simulink model "DroneSimulation"  (R2024a)
settings: Solver=VariableStepAuto  StartTime=0.0  StopTime=100  MaxStep=1e-4  MinStep=1e-6  RelTol=1e-3
undefined symbols (not defined in the file or in its folder): crot, d, g, gustX, gustY, gustZ, I, I_inv, IMU, Ix, Iy, Iz, ks, kt, l, m, ms_mat_inv, pitch_max, rho, roll_max, w_max, windX, windY, windZ, X, Y, Z
libraries: sm_lib x25, nesl_utility x14, simulink x11, slctrl_autotuning x8, mpclib x1, matrix_library x1
(part 1 of 3)
settings Model: SimulationMode=accelerator  Creator=OBWELUC  LastModifiedBy=OBWELUC
settings RTWCC: GPUComputeCapability=3.5
settings ExplorerConfigSet: InternalSimMechanicsExplorerSettings="<ExplorerConfiguration><canonicalview>default</canonicalview><AnimationSetting><BasePlaybackSpeed>1.0</BasePlaybackSpeed><PlaybackSpeedFactor>1.0</PlaybackSpeedFactor></AnimationSetting><TilePanel><TileInfo><Tiles Columns=\"2\" Count=\"4\" Rows=\"2\"><Column Weight=\"0.5\"/><Column Weight=\"0.5\"/><Row Weight=\"0.5\"/><Row Weight=\"0.5\"/><Tile Height=\"1\" Width=\"1\" X=\"0\" Y=\"0\"/><Tile Height=\"1\" Width=\"1\" X=\"0\" Y=\"1\"/><Tile Height=\"1\" Width=\"1\" X=\"1\" Y=\"0\"/><Tile Height=\"1\" Width=\"1\" X=\"1\" Y=\"1\"/></Tiles></TileInfo><SceneInfo><SceneViewer><BGColor><R>0</R><G>0.60000002384185791</G><B>1</B></BGColor><Camera><DoPerspective>off</DoPerspective><Position><X>-0.126727844040819326</X><Y>-7.10861089777495625</Y><Z>0.564557807287776714</Z></Position><Center><X>-0.126727844040819326</X><Y>1.66442092997096287e-07</Y><Z>0.564557807287776714</Z></Center><Up><X>0</X><Y>-0</Y><Z>1</Z></Up><ViewLimDist>1</ViewLimDist><YLim>0.592155844887899185</YLim><XLim>1.20086496625296957</XLim></Camera></SceneViewer><SceneViewer><BGColor><R>0</R><G>0.60000002384185791</G><B>1</B></BGColor><Camera><DoPerspective>off</DoPerspective><Position><X>-0.0834409949380843785</X><Y>0.128196391023159995</Y><Z>6.64461915986203699</Z></Position><Center><X>-0.0834409949380843785</X><Y>0.128196391023159995</Y><Z>-0.000826375150197122821</Z></Center><Up><X>0</X><Y>1</Y><Z>-0</Z></Up><ViewLimDist>1</ViewLimDist><YLim>1.06033933028744309</YLim><XLim>2.1503196583719939</XLim></Camera></SceneViewer><SceneViewer><BGColor><R>0</R><G>0.60000002384185791</G><B>1</B></BGColor><Camera><DoPerspective>off</DoPerspective><Position><X>7.10861089448633621</X><Y>0.203267557456647152</Y><Z>0.620697073756145024</Z></Position><Center><X>-3.2395406890373124e-07</X><Y>0.203267557456647152</Y><Z>0.620697073756145024</Z></Center><Up><X>-0</X><Y>0</Y><Z>1</Z></Up><ViewLimDist>1</ViewLimDist><YLim>0.63905302021013588</YLim><XLim>1.29597029257354102</XLim></Camera></SceneViewer><SceneViewer><BGColor><R>0</R><G>0.60000002384185791</G><B>1</B></BGColor><Camera><DoPerspective>off</DoPerspective><Position><X>4.87676778458632754</X><Y>-4.76365474719023041</Y><Z>1.81715889286770405</Z></Position><Center><X>-0.476731396941828978</X><Y>0.432045443382936933</Y><Z>0.387933409665207618</Z></Center><Up><X>-0.133906028563009039</X><Y>0.132192075511948781</Y><Z>0.982137684179934967</Z></Up><ViewLimDist>1</ViewLimDist><YLim>1.82629377901128631</YLim><XLim>3.70364024307752571</XLim></Camera></SceneViewer></SceneInfo></TilePanel><MechEditorPanel><Cameras/><GfxPanelCameraMap/><VideoCreator><PlaybackSpeedRatio>1.2</PlaybackSpeedRatio><FrameRate>60</FrameRate><VideoFormat>MPEG-4</VideoFormat><FrameSize>[1280 720]</FrameSize></VideoCreator></MechEditorPanel></ExplorerConfiguration>"

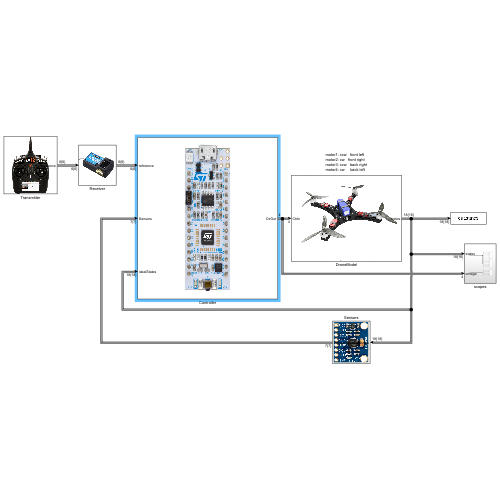
[thumbnail: Simulink's stored preview of the top-level diagram]
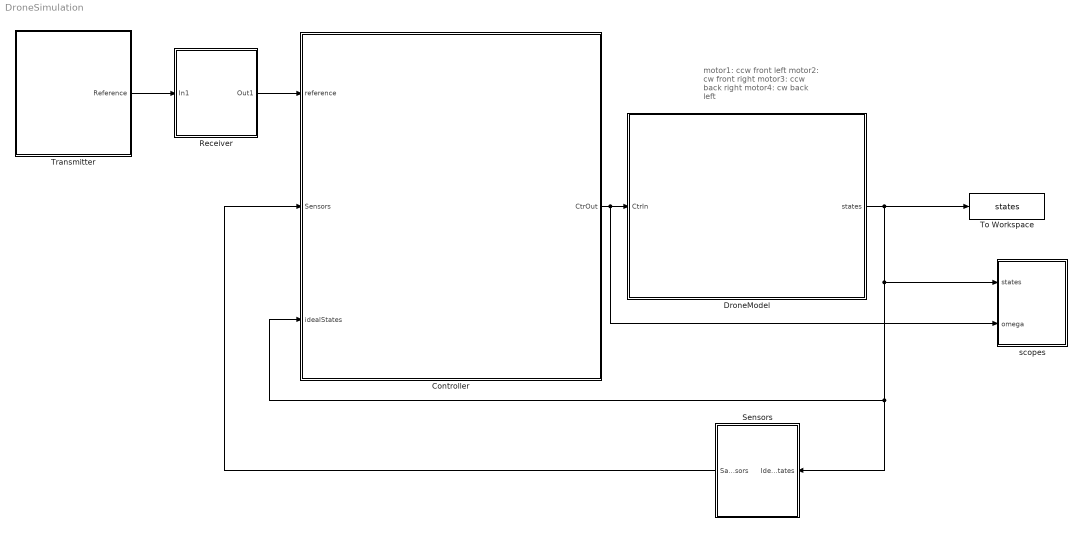
== system DroneSimulation ==
  note: motor1: ccw   front left
      | motor2: cw   front right
      | motor3: ccw   back right
      | motor4: cw     back left
  Controller : Subsystem
      mask Display: image('MFG_NUCLEO-L412KB.jpg');
  DroneModel : Subsystem
      mask Display: image('Assembly2.png');
  Receiver : Subsystem
      mask Display: image('$imagefile'); % Use "Edit Image" on toolstrip to change.
  Sensors : Subsystem
      mask Display: image('$imagefile'); % Use "Edit Image" on toolstrip to change.
  To Workspace : ToWorkspace  VariableName=states  SaveFormat=Timeseries  SampleTime=0.001
  Transmitter : Subsystem
      mask Display: image('$imagefile'); % Use "Edit Image" on toolstrip to change.
  scopes : Subsystem
  wires:
  DroneModel/1(states) -> To Workspace/1, scopes/1(states), Controller/3(idealStates), Sensors/1(IdealStates)
  Controller/1(CtrOut) -> scopes/2(omega), DroneModel/1(CtrIn)
  Transmitter/1(Reference) -> Receiver/1(In1)
  Receiver/1(Out1) -> Controller/1(reference)
  Sensors/1(SampeldSensors) -> Controller/2(Sensors)

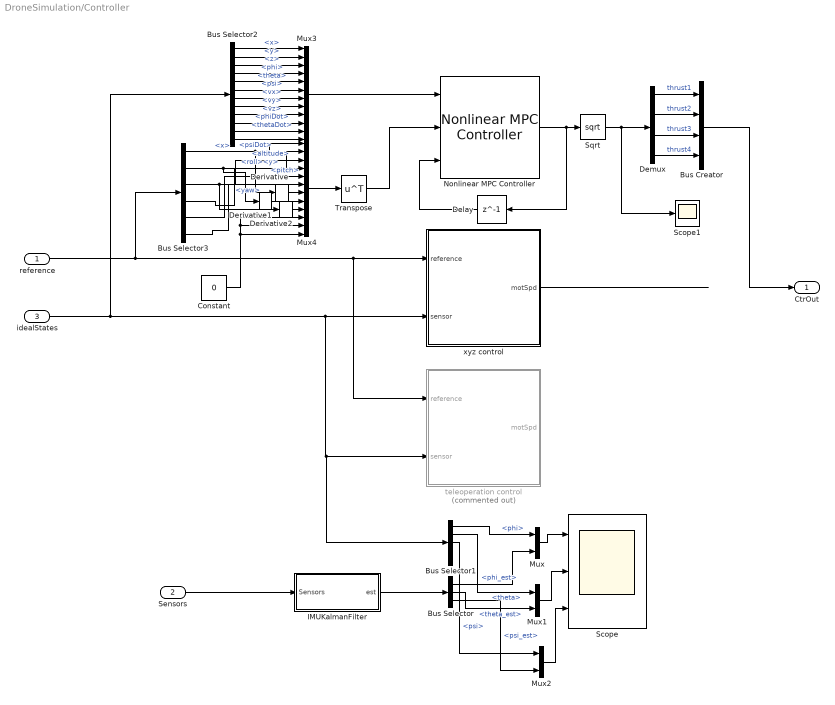
== system DroneSimulation/Controller ==
  reference : Inport
  Sensors : Inport  Port=2
  idealStates : Inport  Port=3
  Bus Creator : BusCreator  Inputs=4
  Bus Selector : BusSelector  OutputSignals=phi_est,theta_est,psi_est
  Bus Selector1 : BusSelector  OutputSignals=phi,theta,psi,ax,ay
  Bus Selector2 : BusSelector  OutputSignals=x,y,z,phi,theta,psi,vx,vy,vz,phiDot,thetaDot,psiDot
  Bus Selector3 : BusSelector  OutputSignals=x,y,altitude,roll,pitch,yaw
  Constant : Constant  Value=0
  Delay : Delay  DelayLength=1
  Demux : Demux
  Derivative : Derivative
  Derivative1 : Derivative
  Derivative2 : Derivative
  IMUKalmanFilter : Subsystem
  Mux : Mux  Inputs=2
  Mux1 : Mux  Inputs=2
  Mux2 : Mux  Inputs=2
  Mux3 : Mux  Inputs=12
  Mux4 : Mux  Inputs=12
  Nonlinear MPC Controller : mpclib/Nonlinear MPC Controller  nlmpcobj=nlmpcobj  UseObjectTs=on  UseMEX=off  md_enabled=off  mvtarget_enabled=off  param_enabled=off  cost_enabled=off  mvseq_enabled=off  stateseq_enabled=off  ovseq_enabled=off  slack_enabled=off  status_enabled=off  ov_min=off  ov_max=off  mv_min=off  mv_max=off  mvrate_min=off  mvrate_max=off  state_min=off  state_max=off  ov_weight=off  mv_weight=off  mvrate_weight=off  ecr_weight=off  nlp_initialize=off
  Scope : Scope  NumInputPorts=3
  Scope1 : Scope
  Sqrt : Sqrt
  Transpose : Math  Operator=transpose
  teleoperation control : Subsystem  Commented=on
  xyz control : Subsystem
  CtrOut : Outport
  wires:
  reference/1 -> Bus Selector3/1, teleoperation control/1(reference), xyz control/1(reference)
  xyz control/1(motSpd) -> ?
  IMUKalmanFilter/1(est) -> Bus Selector/1
  Bus Selector1/1 -> Mux/1  "<phi>"
  Bus Selector/1 -> Mux/2  "<phi_est>"
  Mux/1 -> Scope/1
  Mux1/1 -> Scope/2
  Bus Selector/2 -> Mux1/2  "<theta_est>"
  Bus Selector1/2 -> Mux1/1  "<theta>"
  idealStates/1 -> Bus Selector1/1, teleoperation control/2(sensor), xyz control/2(sensor), Bus Selector2/1
  Sensors/1 -> IMUKalmanFilter/1(Sensors)
  Bus Selector/3 -> Mux2/2  "<psi_est>"
  Bus Selector1/3 -> Mux2/1  "<psi>"
  Mux2/1 -> Scope/3
  Bus Selector2/1 -> Mux3/1  "<x>"
  Bus Selector2/2 -> Mux3/2  "<y>"
  Bus Selector2/3 -> Mux3/3  "<z>"
  Bus Selector2/4 -> Mux3/4  "<phi>"
  Bus Selector2/5 -> Mux3/5  "<theta>"
  Bus Selector2/6 -> Mux3/6  "<psi>"
  Bus Selector2/7 -> Mux3/7  "<vx>"
  Bus Selector2/8 -> Mux3/8  "<vy>"
  Bus Selector2/9 -> Mux3/9  "<vz>"
  Bus Selector2/10 -> Mux3/10  "<phiDot>"
  Bus Selector2/11 -> Mux3/11  "<thetaDot>"
  Bus Selector2/12 -> Mux3/12  "<psiDot>"
  Mux3/1 -> Nonlinear MPC Controller/1
  Mux4/1 -> Transpose/1
  Bus Selector3/1 -> Derivative/1, Mux4/1  "<x>"
  Bus Selector3/2 -> Derivative1/1, Mux4/2  "<y>"
  Bus Selector3/3 -> Derivative2/1, Mux4/3  "<altitude>"
  Constant/1 -> Mux4/12, Mux4/11, Mux4/10
  Bus Selector3/4 -> Mux4/4  "<roll>"
  Bus Selector3/5 -> Mux4/5  "<pitch>"
  Bus Selector3/6 -> Mux4/6  "<yaw>"
  Delay/1 -> Nonlinear MPC Controller/3
  Nonlinear MPC Controller/1 -> Delay/1, Sqrt/1
  Demux/1 -> Bus Creator/1  "thrust1"
  Demux/2 -> Bus Creator/2  "thrust2"
  Demux/3 -> Bus Creator/3  "thrust3"
  Demux/4 -> Bus Creator/4  "thrust4"
  Bus Creator/1 -> CtrOut/1
  Transpose/1 -> Nonlinear MPC Controller/2
  Derivative/1 -> Mux4/7
  Derivative1/1 -> Mux4/8
  Derivative2/1 -> Mux4/9
  Sqrt/1 -> Scope1/1, Demux/1

== system DroneSimulation/DroneModel ==
  CtrIn : Inport
  ComputeThrust : Subsystem
  ComputeTorques : Subsystem
  Dynamics : Subsystem
  visualization : Subsystem
  states : Outport
  wires:
  CtrIn/1 -> ComputeThrust/1(omega), ComputeTorques/1(omega)
  ComputeThrust/1(Fz) -> Dynamics/1(Fz)  "fz"
  Dynamics/1(states) -> visualization/1(states), states/1
  ComputeTorques/1(tau) -> Dynamics/2(tau)  "tau"
  Dynamics/2(t) -> visualization/2(t)
  Dynamics/3(wind) -> visualization/3(wind)

== system DroneSimulation/Receiver ==
  In1 : Inport
  Out1 : Outport
  wires:
  In1/1 -> Out1/1

== system DroneSimulation/Sensors ==
  IdealStates : Inport
  Accelerometer : Subsystem
  Bus Creator : BusCreator  Inputs=3
  barometer : Subsystem
  gyroscope : Subsystem
  SampeldSensors : Outport
  wires:
  IdealStates/1 -> barometer/1(IdealStates), gyroscope/1(IdealStates), Accelerometer/1(IdealStates)
  Bus Creator/1 -> SampeldSensors/1
  Accelerometer/1(accelerometerStates) -> Bus Creator/3  "accelerometer"
  gyroscope/1(gyroscopeStates) -> Bus Creator/2  "gyroscope"
  barometer/1(barometerStates) -> Bus Creator/1  "barometer"

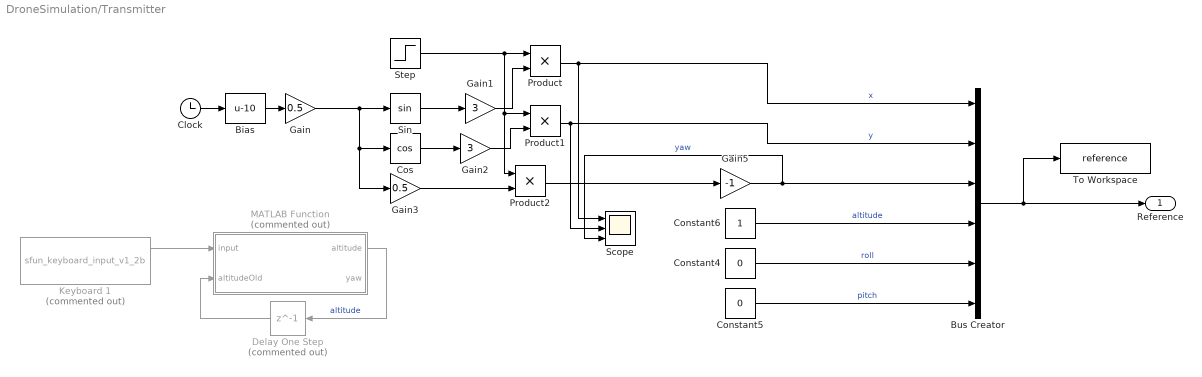
== system DroneSimulation/Transmitter ==
  Bias : Bias  Bias=-10  SaturateOnIntegerOverflow=off
  Bus Creator : BusCreator  Inputs=6
  Clock : Clock
  Constant4 : Constant  Value=0
  Constant5 : Constant  Value=0
  Constant6 : Constant
  Cos : Trigonometry  Operator=cos
  Delay One Step : Delay  Commented=on  DelayLength=1
  Gain : Gain  Gain=0.5
  Gain1 : Gain  Gain=3
  Gain2 : Gain  Gain=3
  Gain3 : Gain  Gain=0.5
  Gain5 : Gain  Gain=-1
  Keyboard 1 : M-S-Function  Commented=on  FunctionName=sfun_keyboard_input_v1_2b  mask(Keyboard Input){}
      mask help: Keyboard Input
      mask Display: fprintf('Keyboard');
  MATLAB Function : MATLAB Function  Commented=on  TreatAsAtomicUnit=on
  Product : Product
  Product1 : Product
  Product2 : Product
  Scope : Scope  NumInputPorts=3
  Sin : Trigonometry
  Step : Step  Time=10  SampleTime=0
  To Workspace : ToWorkspace  VariableName=reference  SaveFormat=Timeseries  SampleTime=0.001
  Reference : Outport
  wires:
  Bus Creator/1 -> To Workspace/1, Reference/1
  Product2/1 -> Gain5/1
  Cos/1 -> Gain2/1
  Sin/1 -> Gain1/1
  MATLAB Function/1(altitude) -> Delay One Step/1  "altitude"
  Constant4/1 -> Bus Creator/5  "roll"
  Constant5/1 -> Bus Creator/6  "pitch"
  Keyboard 1/1 -> MATLAB Function/1(input)
  Delay One Step/1 -> MATLAB Function/2(altitudeOld)
  Constant6/1 -> Bus Creator/4  "altitude"
  Clock/1 -> Bias/1
  Gain/1 -> Gain3/1, Cos/1, Sin/1
  Product/1 -> Scope/1, Bus Creator/1  "x"
  Product1/1 -> Scope/2, Bus Creator/2  "y"
  Gain1/1 -> Product/2
  Step/1 -> Product2/1, Product1/1, Product/1
  Gain2/1 -> Product1/2
  Gain5/1 -> Scope/3, Bus Creator/3  "yaw"
  Gain3/1 -> Product2/2
  Bias/1 -> Gain/1

== system DroneSimulation/scopes ==
  states : Inport
  omega : Inport  Port=2
  Bus Selector : BusSelector  OutputSignals=x,y,z,vx,vy,vz
  Bus Selector1 : BusSelector  OutputSignals=phi,theta,psi,phiDot,thetaDot,psiDot
  Bus Selector2 : BusSelector  OutputSignals=thrust1,thrust2,thrust3,thrust4
  Scope : Scope  NumInputPorts=4
  linearStates : Scope  NumInputPorts=6
  rotationalStates : Scope  NumInputPorts=6
  wires:
  states/1 -> Bus Selector1/1, Bus Selector/1
  Bus Selector1/1 -> rotationalStates/1  "<phi>"
  Bus Selector1/2 -> rotationalStates/2  "<theta>"
  Bus Selector1/3 -> rotationalStates/3  "<psi>"
  Bus Selector1/6 -> rotationalStates/6  "<psiDot>"
  Bus Selector1/4 -> rotationalStates/4  "<phiDot>"
  Bus Selector1/5 -> rotationalStates/5  "<thetaDot>"
  Bus Selector/2 -> linearStates/2  "<y>"
  Bus Selector/1 -> linearStates/1  "<x>"
  Bus Selector/3 -> linearStates/3  "<z>"
  Bus Selector/4 -> linearStates/4  "<vx>"
  Bus Selector/6 -> linearStates/6  "<vz>"
  Bus Selector/5 -> linearStates/5  "<vy>"
  omega/1 -> Bus Selector2/1
  Bus Selector2/1 -> Scope/1  "<thrust1>"
  Bus Selector2/2 -> Scope/2  "<thrust2>"
  Bus Selector2/3 -> Scope/3  "<thrust3>"
  Bus Selector2/4 -> Scope/4  "<thrust4>"

== system DroneSimulation/Controller/IMUKalmanFilter ==
  Sensors : Inport
  Bus Creator : BusCreator  Inputs=3
  Bus Selector : BusSelector  OutputSignals=gyroscope.phid,gyroscope.thetad,gyroscope.psid,accelerometer.ax,accelerometer.ay,accelerometer.az
  Delay One Step : Delay  DelayLength=1  InitialCondition=eye(3)*0.003872  SampleTime=0.001
  Delay One Step1 : Delay  DelayLength=1  InitialCondition=[0;0; 0]  SampleTime=0.001
  Demux : Demux  Outputs=3
  KF : MATLAB Function  TreatAsAtomicUnit=on  SystemSampleTime=0.001
  Mux : Mux  Inputs=6
  est : Outport
  wires:
  Sensors/1 -> Bus Selector/1
  Bus Selector/1 -> Mux/1  "<phid>"
  Bus Selector/2 -> Mux/2  "<thetad>"
  Bus Selector/3 -> Mux/3  "<psid>"
  Bus Selector/4 -> Mux/4  "<ax>"
  Bus Selector/5 -> Mux/5  "<ay>"
  Bus Selector/6 -> Mux/6  "<az>"
  Mux/1 -> KF/1(IMUmeas)
  KF/2(P_p) -> Delay One Step/1
  Delay One Step/1 -> KF/3("P_p ")
  Delay One Step1/1 -> KF/2("xhat ")
  KF/1(xhat) -> Demux/1, Delay One Step1/1
  Demux/1 -> Bus Creator/1  "phi_est"
  Demux/2 -> Bus Creator/2  "theta_est"
  Bus Creator/1 -> est/1
  Demux/3 -> Bus Creator/3  "psi_est"

== system DroneSimulation/Controller/teleoperation control ==
  reference : Inport
  sensor : Inport  Port=2
  MMA : Subsystem
  altitude PID : Subsystem
  pitch PID : Subsystem
  roll PID : Subsystem
  yaw PID : Subsystem
  motSpd : Outport
  wires:
  sensor/1 -> roll PID/2(sensor), pitch PID/2(sensor), yaw PID/2(sensor), altitude PID/2(sensor)
  pitch PID/1(cmd) -> MMA/2(pitch)  "taup"
  roll PID/1(cmd) -> MMA/1(roll)  "taur"
  yaw PID/1(cmd) -> MMA/3(yaw)  "tauy"
  reference/1 -> pitch PID/1(reference), roll PID/1(reference), yaw PID/1(reference), altitude PID/1(reference)
  altitude PID/1(cmd) -> MMA/4(thrust)  "fz"
  MMA/1(motSpd) -> motSpd/1

== system DroneSimulation/Controller/xyz control ==
  reference : Inport
  sensor : Inport  Port=2
  MMA : Subsystem
  altitude PID : Subsystem
  pitch PID : Subsystem
  positionController : Subsystem
  roll PID : Subsystem
  yaw PID : Subsystem
  motSpd : Outport
  wires:
  sensor/1 -> positionController/2(sensor), roll PID/2(sensor), pitch PID/2(sensor), yaw PID/2(sensor), altitude PID/2(sensor)
  pitch PID/1(cmd) -> MMA/2(pitch)  "taup"
  positionController/1(rollRef) -> roll PID/1(reference)
  roll PID/1(cmd) -> MMA/1(roll)  "taur"
  reference/1 -> positionController/1(reference), yaw PID/1(reference), altitude PID/1(reference)
  yaw PID/1(cmd) -> MMA/3(yaw)  "tauy"
  positionController/2(pitchRef) -> pitch PID/1(reference)
  altitude PID/1(cmd) -> MMA/4(thrust)  "fz"
  MMA/1(motSpd) -> motSpd/1

== system DroneSimulation/DroneModel/ComputeThrust ==
  omega : Inport
  Demux : Demux
  Gain : Gain  Gain=kt
  Square{,1..3} (4 alike) : Math  Operator=square
  Sum : Sum  Inputs=|++++
  Fz : Outport
  wires:
  Square3/1 -> Sum/4
  Square/1 -> Sum/1
  Square1/1 -> Sum/2
  Square2/1 -> Sum/3
  Sum/1 -> Gain/1
  Gain/1 -> Fz/1
  omega/1 -> Demux/1
  Demux/1 -> Square/1
  Demux/2 -> Square1/1
  Demux/3 -> Square2/1
  Demux/4 -> Square3/1

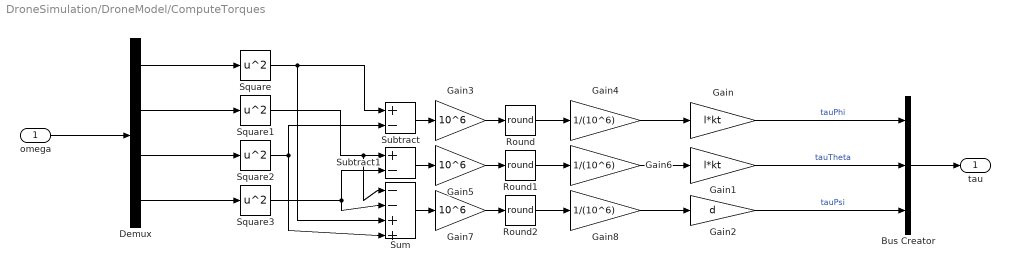
== system DroneSimulation/DroneModel/ComputeTorques ==
  omega : Inport
  Bus Creator : BusCreator  Inputs=3
  Demux : Demux
  Gain : Gain  Gain=l*kt
  Gain1 : Gain  Gain=l*kt
  Gain2 : Gain  Gain=d
  Gain3 : Gain  Gain=10^6
  Gain4 : Gain  Gain=1/(10^6)
  Gain5 : Gain  Gain=10^6
  Gain6 : Gain  Gain=1/(10^6)
  Gain7 : Gain  Gain=10^6
  Gain8 : Gain  Gain=1/(10^6)
  Round : Rounding  Operator=round
  Round1 : Rounding  Operator=round
  Round2 : Rounding  Operator=round
  Square{,1..3} (4 alike) : Math  Operator=square  OutDataTypeStr=double
  Subtract : Sum  Inputs=+-
  Subtract1 : Sum  Inputs=+-
  Sum : Sum  Inputs=|--++
  tau : Outport
  wires:
  Demux/1 -> Square/1
  Demux/4 -> Square3/1
  Demux/3 -> Square2/1
  Demux/2 -> Square1/1
  Square1/1 -> Sum/1, Subtract1/1
  Square3/1 -> Sum/2, Subtract1/2
  Subtract/1 -> Gain3/1
  Gain/1 -> Bus Creator/1  "tauPhi"
  Square2/1 -> Subtract/2, Sum/4
  Square/1 -> Subtract/1, Sum/3
  Subtract1/1 -> Gain5/1
  Gain1/1 -> Bus Creator/2  "tauTheta"
  Sum/1 -> Gain7/1
  Gain2/1 -> Bus Creator/3  "tauPsi"
  Bus Creator/1 -> tau/1
  omega/1 -> Demux/1
  Gain3/1 -> Round/1
  Round/1 -> Gain4/1
  Gain4/1 -> Gain/1
  Gain5/1 -> Round1/1
  Round1/1 -> Gain6/1
  Gain6/1 -> Gain1/1
  Gain7/1 -> Round2/1
  Round2/1 -> Gain8/1
  Gain8/1 -> Gain2/1

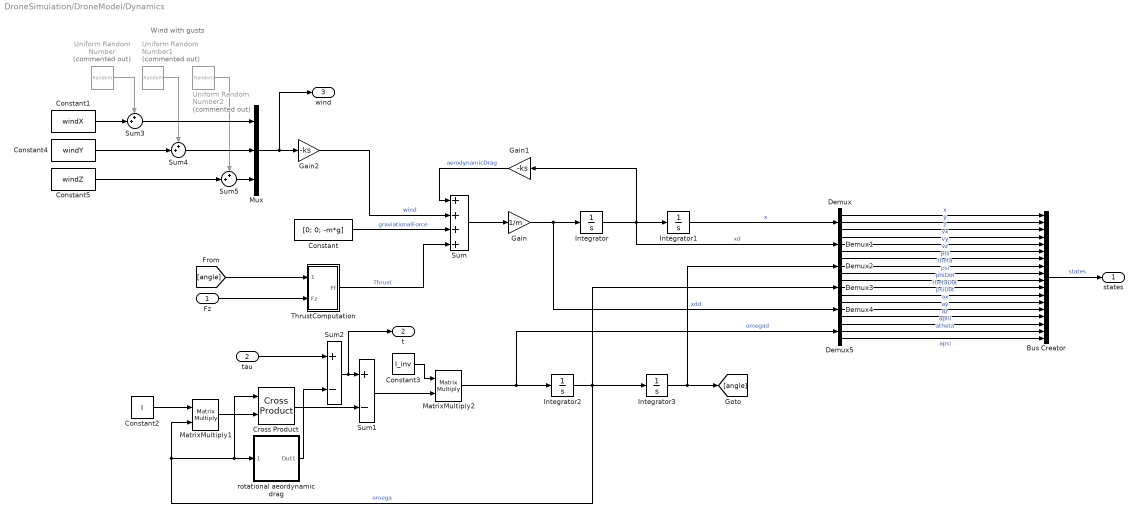
== system DroneSimulation/DroneModel/Dynamics ==
  note: Wind with gusts
  Fz : Inport
  tau : Inport  Port=2
  Bus Creator : BusCreator  Inputs=18
  Constant : Constant  Value=[0; 0; -m*g]
  Constant1 : Constant  Value=windX
  Constant2 : Constant  Value=I
  Constant3 : Constant  Value=I_inv
  Constant4 : Constant  Value=windY
  Constant5 : Constant  Value=windZ
  Cross Product : matrix_library/Cross Product
  Demux{,1..5} (6 alike) : Demux  Outputs=3
  Gain : Gain  Gain=1/m
  Gain1 : Gain  Gain=-ks
  Gain2 : Gain  Gain=-ks
  Integrator{,1..3} (4 alike) : Integrator
  MatrixMultiply1 : Product  Multiplication=Matrix(*)
  MatrixMultiply2 : Product  Multiplication=Matrix(*)
  Mux : Mux  Inputs=3
  Sum : Sum  Inputs=++++
  Sum1 : Sum  Inputs=+-
  Sum2 : Sum  Inputs=+-
  Sum3 : Sum  Inputs=++|
  Sum4 : Sum  Inputs=++|
  Sum5 : Sum  Inputs=++|
  ThrustComputation : Subsystem
  Uniform Random Number : UniformRandomNumber  Commented=on  Minimum=-gustX  Maximum=gustX  SampleTime=1
  Uniform Random Number1 : UniformRandomNumber  Commented=on  Minimum=-gustY  Maximum=gustY  Seed=2  SampleTime=1
  Uniform Random Number2 : UniformRandomNumber  Commented=on  Minimum=-gustZ  Maximum=gustZ*0  Seed=1  SampleTime=1
  rotational aeordynamic drag : Subsystem
  states : Outport
  t : Outport  Port=2
  wind : Outport  Port=3
  wires:
  tau/1 -> Sum2/1
  Gain/1 -> Demux4/1, Integrator/1  "xdd"
  Integrator/1 -> Gain1/1, Demux1/1, Integrator1/1  "xd"
  Bus Creator/1 -> states/1  "states"
  Constant/1 -> Sum/3  "graviationalForce"
  Gain1/1 -> Sum/1  "aerodynamicDrag"
  Sum/1 -> Gain/1
  MatrixMultiply2/1 -> Demux5/1, Integrator2/1  "omegad"
  Integrator2/1 -> MatrixMultiply1/2, Cross Product/1, rotational aeordynamic drag/1(omega), Demux3/1, Integrator3/1  "omega"
  MatrixMultiply1/1 -> Cross Product/2
  Constant2/1 -> MatrixMultiply1/1
  Cross Product/1 -> Sum1/2
  Sum1/1 -> MatrixMultiply2/2
  Constant3/1 -> MatrixMultiply2/1
  Integrator3/1 -> Demux2/1, [angle]
  Integrator1/1 -> Demux/1  "x"
  Demux/1 -> Bus Creator/1  "x"
  Demux/2 -> Bus Creator/2  "y"
  Demux/3 -> Bus Creator/3  "z"
  Demux1/1 -> Bus Creator/4  "vx"
  Demux1/2 -> Bus Creator/5  "vy"
  Demux1/3 -> Bus Creator/6  "vz"
  Demux2/1 -> Bus Creator/7  "phi"
  Demux2/2 -> Bus Creator/8  "theta"
  Demux2/3 -> Bus Creator/9  "psi"
  Demux3/1 -> Bus Creator/10  "phiDot"
  Demux3/2 -> Bus Creator/11  "thetaDot"
  Demux3/3 -> Bus Creator/12  "psiDot"
  rotational aeordynamic drag/1(Out1) -> Sum2/2
  Fz/1 -> ThrustComputation/2(Fz)
  ThrustComputation/1(Ff) -> Sum/4  "Thrust"
  [angle] -> ThrustComputation/1(Angle)
  Demux4/1 -> Bus Creator/13  "ax"
  Demux4/2 -> Bus Creator/14  "ay"
  Demux5/1 -> Bus Creator/16  "aphi"
  Demux5/2 -> Bus Creator/17  "atheta"
  Demux5/3 -> Bus Creator/18  "apsi"
  Sum2/1 -> t/1, Sum1/1
  Uniform Random Number/1 -> Sum3/1
  Uniform Random Number1/1 -> Sum4/1
  Uniform Random Number2/1 -> Sum5/1
  Mux/1 -> wind/1, Gain2/1
  Gain2/1 -> Sum/2  "wind"
  Sum3/1 -> Mux/1
  Constant1/1 -> Sum3/2
  Sum4/1 -> Mux/2
  Constant4/1 -> Sum4/2
  Sum5/1 -> Mux/3
  Constant5/1 -> Sum5/2
  Demux4/3 -> Bus Creator/15  "az"
